simulink model "bracket_simulink_model"  (R2024b)
settings: Solver=FixedStepAuto  StartTime=0.0  StopTime=2.5  FixedStep=0.01  RelTol=1e-3
values from neighbouring files (symbols this model uses):
  c = 66.6    [bracket.m]
  k = 20000    [bracket.m]
  m = 2.22    [bracket.m]
settings Model: Creator=DELL  LastModifiedBy=DELL
settings DataIOCC: ReturnWorkspaceOutputs=off

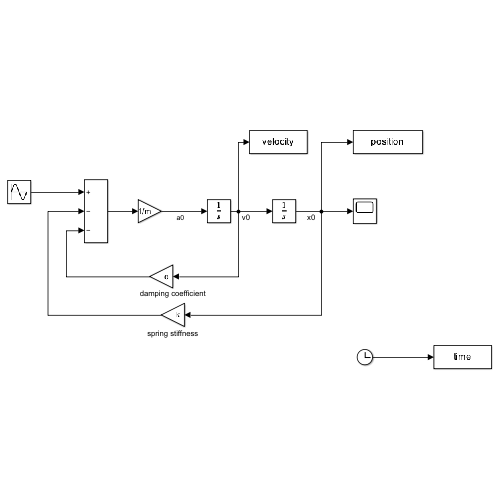
[thumbnail: Simulink's stored preview of the top-level diagram]
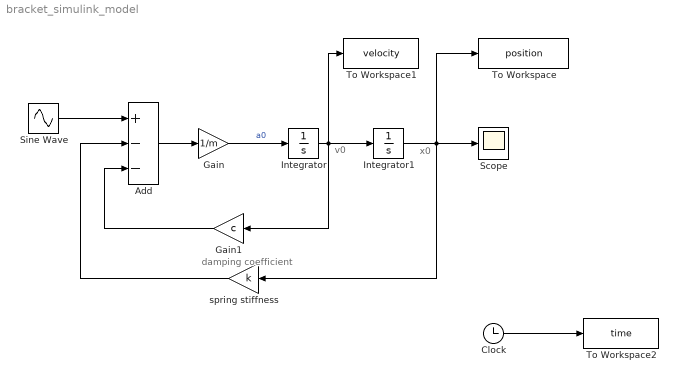
== system bracket_simulink_model ==
  note: damping coefficient
  note: x0
  note: v0
  Add : Sum  Inputs=+--
  Clock : Clock
  Gain : Gain  Gain=1/m
  Gain1 : Gain  Gain=c
  Integrator : Integrator
  Integrator1 : Integrator
  Scope : Scope
  Sine Wave : Sin  Amplitude=100  Frequency=125.66  SampleTime=0
  To Workspace : ToWorkspace  VariableName=position  SampleTime=-1
  To Workspace1 : ToWorkspace  VariableName=velocity  SampleTime=-1
  To Workspace2 : ToWorkspace  VariableName=time  SampleTime=-1
  spring stiffness : Gain  Gain=k
  wires:
  Sine Wave/1 -> Add/1
  Gain/1 -> Integrator/1  "a0"
  Add/1 -> Gain/1
  Integrator/1 -> To Workspace1/1, Gain1/1, Integrator1/1
  Integrator1/1 -> Scope/1, To Workspace/1, spring stiffness/1
  Gain1/1 -> Add/3
  spring stiffness/1 -> Add/2
  Clock/1 -> To Workspace2/1
